simulink library "lib_beam"  (R2020b)
settings: Solver=VariableStepAuto  StartTime=0.0  StopTime=10.0  RelTol=1e-3
settings Model: Creator=hao  LastModifiedBy=hao

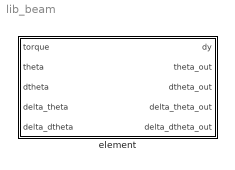
== system lib_beam ==
  element : Subsystem  mask{IA=0, k1=0, k2=0, k3=0, b=0, ElementLength=0}
      mask prompts: IA "inertial"; k1 "spring coefficient1"; k2 "spring coefficient2"; k3 "spring coefficient3"; b "damper coefficient"; ElementLength "length"

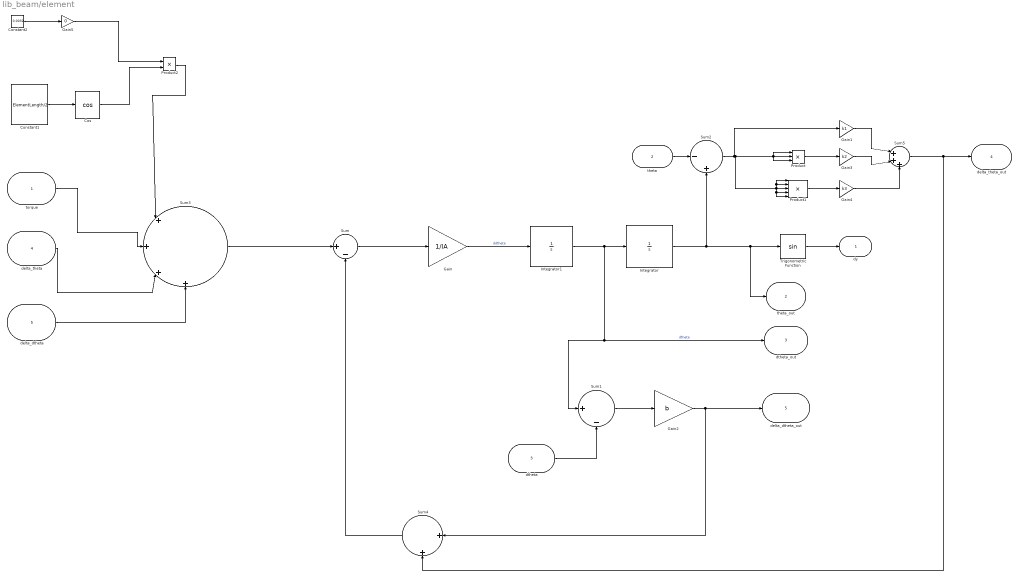
== system lib_beam/element ==
  torque : Inport
  theta : Inport  Port=2
  dtheta : Inport  Port=3
  delta_theta : Inport  Port=4
  delta_dtheta : Inport  Port=5
  Constant1 : Constant  Value=ElementLength/2
  Constant2 : Constant  Value=0.0032
  Cos : Trigonometry  Operator=cos
  Gain : Gain  Gain=1/IA
  Gain1 : Gain  Gain=k1
  Gain2 : Gain  Gain=b
  Gain3 : Gain  Gain=k2
  Gain4 : Gain  Gain=k3
  Gain5 : Gain  Gain=0
  Integrator : Integrator
  Integrator1 : Integrator
  Product : Product  Inputs=3
  Product1 : Product  Inputs=5
  Product2 : Product
  Sum : Sum  Inputs=|+-
  Sum1 : Sum  Inputs=|+-
  Sum2 : Sum  Inputs=|-+
  Sum3 : Sum  Inputs=|++++
  Sum4 : Sum  Inputs=|++
  Sum5 : Sum  Inputs=|+++
  Trigonometric Function : Trigonometry
  dy : Outport
  theta_out : Outport  Port=2
  dtheta_out : Outport  Port=3
  delta_theta_out : Outport  Port=4
  delta_dtheta_out : Outport  Port=5
  wires:
  Sum1/1 -> Gain2/1
  dtheta/1 -> Sum1/2
  Sum/1 -> Gain/1
  delta_dtheta/1 -> Sum3/4
  Integrator/1 -> Trigonometric Function/1, theta_out/1, Sum2/2
  Sum3/1 -> Sum/1
  theta/1 -> Sum2/1
  Gain/1 -> Integrator1/1  "ddtheta"
  Integrator1/1 -> dtheta_out/1, Sum1/1, Integrator/1  "dtheta"
  Gain2/1 -> delta_dtheta_out/1, Sum4/1
  Sum5/1 -> delta_theta_out/1, Sum4/2
  Sum4/1 -> Sum/2
  Trigonometric Function/1 -> dy/1
  Gain1/1 -> Sum5/1
  Gain3/1 -> Sum5/2
  Gain4/1 -> Sum5/3
  Product/1 -> Gain3/1
  Sum2/1 -> Product/2, Product/3, Product/1, Product1/1, Product1/2, Product1/4, Product1/5, Product1/3, Gain1/1
  Product1/1 -> Gain4/1
  Constant1/1 -> Cos/1
  Cos/1 -> Product2/2
  delta_theta/1 -> Sum3/3
  torque/1 -> Sum3/2
  Product2/1 -> Sum3/1
  Constant2/1 -> Gain5/1
  Gain5/1 -> Product2/1
